simulink model "lowwind"  (Simulink 8.0)
settings: Solver=ode45  StartTime=0.0  StopTime=300.0  RelTol=1e-3
undefined symbols (not defined in the file or in its folder): ctrlpara, Exp_Lamda, Jg, Jr, Kt, ng, R
libraries: simulink_need_slupdate x1, wt_blockset_v3 x1
settings Model: Creator=acer  LastModifiedBy=Administrator
settings DataIOCC: SignalLoggingSaveFormat=ModelDataLogs
settings DebuggingCC: FcnCallInpInsideContextMsg=UseLocalSettings  StrictBusMsg=Warning
settings GRTTargetCC: CombineOutputUpdateFcns=off  GRTInterface=on

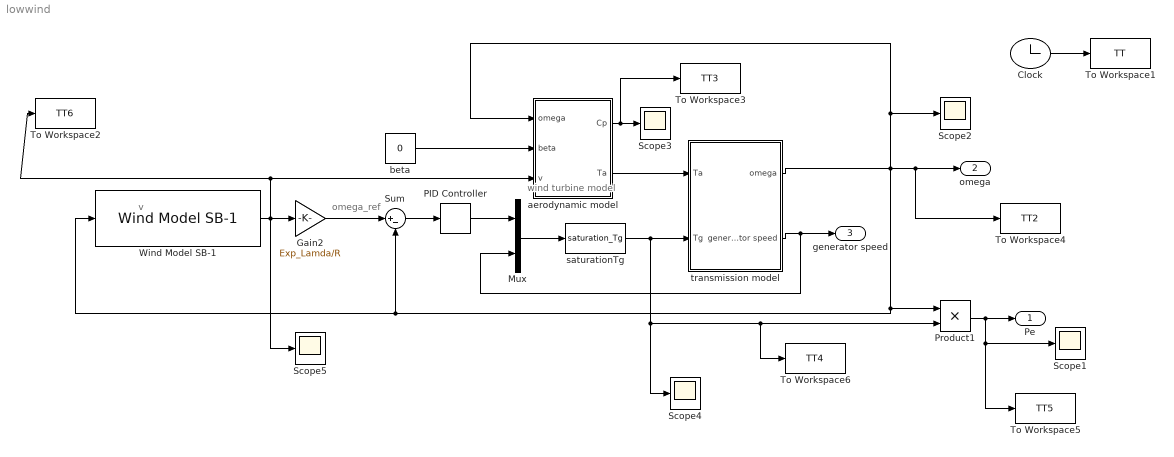
== system lowwind ==
  note: v
  note: wind turbine model
  note: omega_ref
  Clock : Clock
  Gain2 : Gain  Gain=Exp_Lamda/R
  Mux : Mux  Inputs=2
  PID Controller : simulink_need_slupdate/PID Controller  P=ctrlpara(1)  I=ctrlpara(2)  D=0
  Product1 : Product  RndMeth=Zero
  Scope{1..5} (5 alike) : Scope
      Scope1 settings: TimeRange=120  YMin=300000  YMax=750000
      Scope2 settings: TimeRange=120  YMin=0.425  YMax=0.4345
      Scope3 settings: TimeRange=120  YMin=0.31  YMax=0.5  SaveName=ScopeData2
      Scope4 settings: TimeRange=120  YMin=0.31  YMax=0.5  SaveName=ScopeData3
      Scope5 settings: TimeRange=120  YMin=0.31  YMax=0.5  SaveName=ScopeData4
  Sum : Sum  Inputs=|+-
  To Workspace1 : ToWorkspace  VariableName=TT  SampleTime=-1
  To Workspace2 : ToWorkspace  VariableName=TT6  SampleTime=-1
  To Workspace3 : ToWorkspace  VariableName=TT3  SampleTime=-1
  To Workspace4 : ToWorkspace  VariableName=TT2  SampleTime=-1
  To Workspace5 : ToWorkspace  VariableName=TT5  SampleTime=-1
  To Workspace6 : ToWorkspace  VariableName=TT4  SampleTime=-1
  Wind Model SB-1 : wt_blockset_v3/Mechanical Components/Wind Model SB-1  D_rotor=72  v_mean=9  roughness=100  turb_int=12  T_sample=1
  aerodynamic model : Subsystem
  beta : Constant  Value=0
  saturationTg : MATLABFcn  MATLABFcn=saturation_Tg
  transmission model : Subsystem
  Pe : Outport
  omega : Outport  Port=2
  generator speed : Outport  Port=3
  wires:
  Sum/1 -> PID Controller/1
  Gain2/1 -> Sum/1
  Product1/1 -> Pe/1, Scope1/1, To Workspace5/1
  transmission model/2(generator speed) -> generator speed/1, Mux/2
  Wind Model SB-1/1 -> Gain2/1, aerodynamic model/3(v), To Workspace2/1, Scope5/1
  PID Controller/1 -> Mux/1
  transmission model/1(omega) -> aerodynamic model/1(omega), Scope2/1, Sum/2, Wind Model SB-1/1, Product1/1, omega/1, To Workspace4/1
  Clock/1 -> To Workspace1/1
  beta/1 -> aerodynamic model/2(beta)
  aerodynamic model/1(Cp) -> Scope3/1, To Workspace3/1
  aerodynamic model/2(Ta) -> transmission model/1(Ta)
  Mux/1 -> saturationTg/1
  saturationTg/1 -> transmission model/2(Tg), Scope4/1, Product1/2, To Workspace6/1

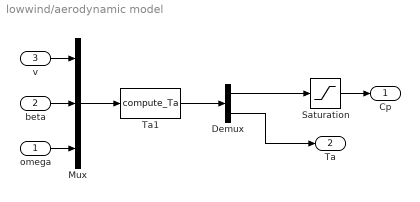
== system lowwind/aerodynamic model ==
  omega : Inport
  beta : Inport  Port=2
  v : Inport  Port=3
  Demux : Demux  Outputs=2
  Mux : Mux  Inputs=3
  Saturation : Saturate  UpperLimit=0.442
  Ta1 : MATLABFcn  MATLABFcn=compute_Ta
  Cp : Outport
  Ta : Outport  Port=2
  wires:
  Mux/1 -> Ta1/1
  v/1 -> Mux/1
  beta/1 -> Mux/2
  omega/1 -> Mux/3
  Ta1/1 -> Demux/1
  Demux/1 -> Saturation/1
  Demux/2 -> Ta/1
  Saturation/1 -> Cp/1

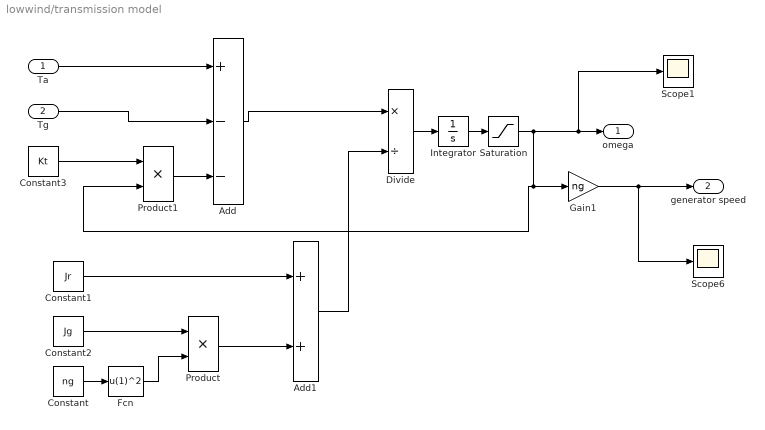
== system lowwind/transmission model ==
  Ta : Inport
  Tg : Inport  Port=2
  Add : Sum  Inputs=+--
  Add1 : Sum
  Constant : Constant  Value=ng
  Constant1 : Constant  Value=Jr
  Constant2 : Constant  Value=Jg
  Constant3 : Constant  Value=Kt  VectorParams1D=off
  Divide : Product  Inputs=*/
  Fcn : Fcn  Expr=u(1)^2
  Gain1 : Gain  Gain=ng
  Integrator : Integrator  InitialCondition=1.12
  Product : Product  RndMeth=Zero
  Product1 : Product  RndMeth=Zero
  Saturation : Saturate  UpperLimit=1.97
  Scope1 : Scope
      settings: TimeRange=80  YMin=0.9  YMax=1.65  SaveName=ScopeData9
  Scope6 : Scope
      settings: TimeRange=80  YMin=70  YMax=155  SaveName=ScopeData5
  omega : Outport
  generator speed : Outport  Port=2
  wires:
  Fcn/1 -> Product/2
  Constant/1 -> Fcn/1
  Ta/1 -> Add/1
  Constant2/1 -> Product/1
  Constant1/1 -> Add1/1
  Product/1 -> Add1/2
  Add/1 -> Divide/1
  Add1/1 -> Divide/2
  Divide/1 -> Integrator/1
  Integrator/1 -> Saturation/1
  Gain1/1 -> generator speed/1, Scope6/1
  Product1/1 -> Add/3
  Constant3/1 -> Product1/1
  Tg/1 -> Add/2
  Saturation/1 -> Gain1/1, Product1/2, omega/1, Scope1/1
